simulink model "simPodB"  (R2024b)
settings: Solver=VariableStepAuto  StartTime=0.0  StopTime=10.0  RelTol=1e-3
values from neighbouring files (symbols this model uses):
  B = 20    [mFilePodA.m]    (also in mFilePodB.m)
  g = 9.81    [mFilePodA.m]    (also in mFilePodB.m)
  k = 200    [mFilePodA.m]    (also in mFilePodB.m)
  M = 10    [mFilePodA.m]    (also in mFilePodB.m)
settings Model: Creator=Ishak  LastModifiedBy=Ishak

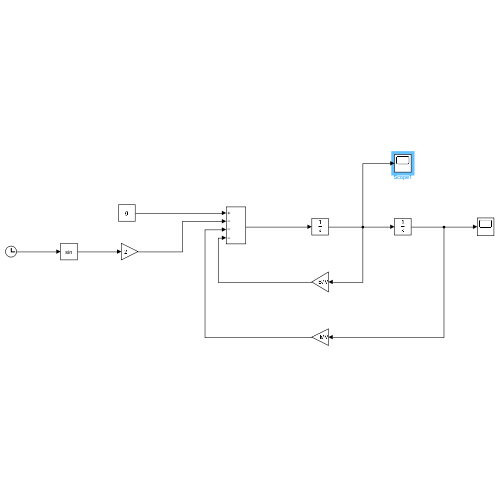
[thumbnail: Simulink's stored preview of the top-level diagram]
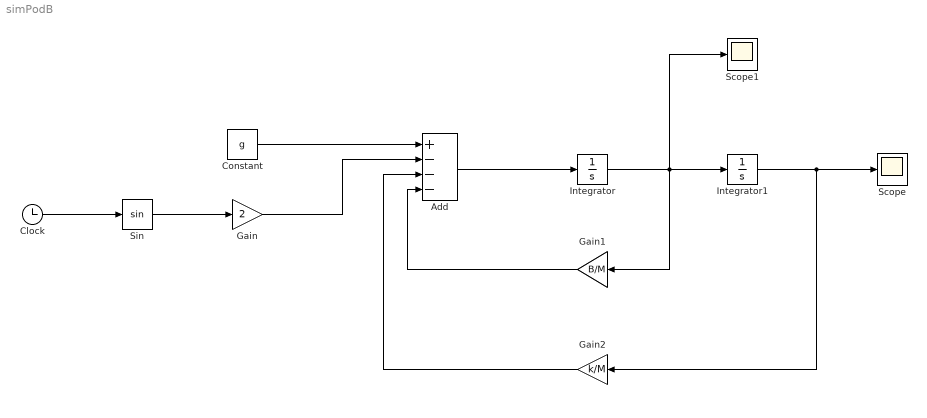
== system simPodB ==
  Add : Sum  Inputs=+---
  Clock : Clock
  Constant : Constant  Value=g
  Gain : Gain  Gain=2
  Gain1 : Gain  Gain=B/M
  Gain2 : Gain  Gain=k/M
  Integrator : Integrator
  Integrator1 : Integrator
  Scope : Scope
  Scope1 : Scope
  Sin : Trigonometry
  wires:
  Integrator/1 -> Scope1/1, Gain1/1, Integrator1/1
  Integrator1/1 -> Gain2/1, Scope/1
  Add/1 -> Integrator/1
  Constant/1 -> Add/1
  Clock/1 -> Sin/1
  Sin/1 -> Gain/1
  Gain/1 -> Add/2
  Gain1/1 -> Add/4
  Gain2/1 -> Add/3
